simulink model "HVDCMTGW"  (R2025b)
settings: Solver=VariableStepAuto  StartTime=0.0  StopTime=Tsim  FixedStep=5e-5  RelTol=1e-3
PreLoadFcn:
  | SimulationTime = 3.5;
  | HVDCParameters;
  | Tsim = 3.5;
undefined symbols (not defined in the file): base, Base, Connection1, Connection2, Connection3, DiscIntNeverNeededParam, ee_sli_rtmsupport, frt, gcbh, grid, HVDC, lvrt, onshoreGfm, pll, pmsm, PVController, time, Ts, windController, windTransformer, windTurbine
libraries: fl_lib x51, ee_lib x46, nesl_utility x41, simulink x18, eeGeneralControl x12, eeTransforms x6
(part 4 of 4)

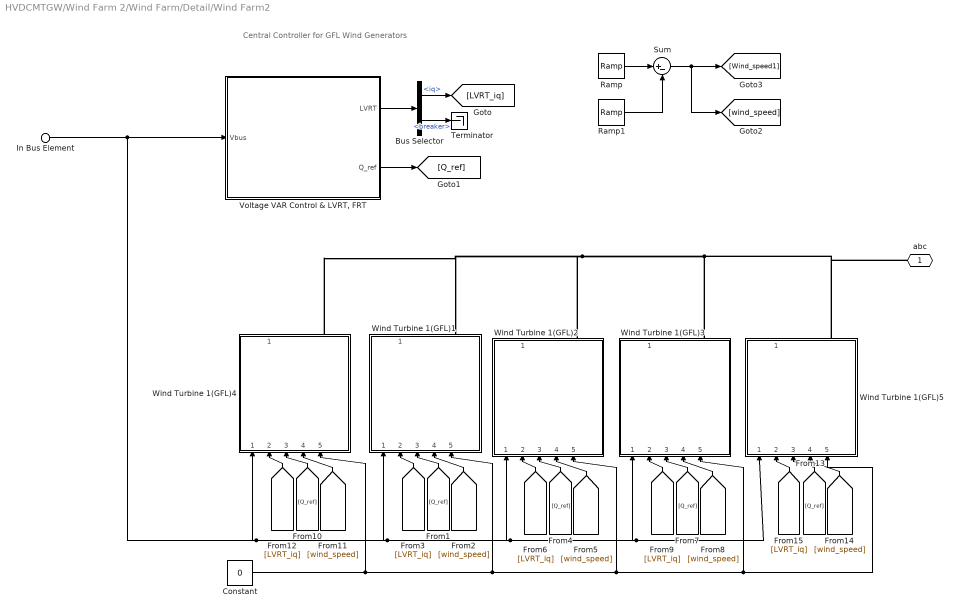
== system HVDCMTGW/Wind Farm 2/Wind Farm/Detail/Wind Farm2 ==
  note: Central Controller for GFL Wind Generators
  In Bus Element : Inport  PortName=Vbus
  Bus Selector : BusSelector  OutputSignals=iq,breaker
  Constant : Constant  Value=0
  Ramp : simulink/Sources/Ramp  slope=-3  start=time.renewablevariation  InitialOutput=11
  Ramp1 : simulink/Sources/Ramp  slope=-3  start=time.renewablevariation+0.2  InitialOutput=0
  Sum : Sum  Inputs=|+-
  Terminator : Terminator
  "Voltage VAR Control & LVRT, FRT" : Subsystem
      mask Display: image('$imagefile'); % Use "Edit Image" on toolstrip to change.
  Wind Turbine 1(GFL){1..5} (5 alike) : Subsystem  ReferencedSubsystem=WindGFLMpp  p=pmsm.p  psim=pmsm.psim  Rs=pmsm.rs  Ld=pmsm.ld  Lq=pmsm.lq  Kdip_sm=pmsm.ld*pmsm.alpha  Kdii_sm=pmsm.rs*pmsm.alpha  Kqip_sm=pmsm.lq*pmsm.alpha  Kqii_sm=pmsm.rs*pmsm.alpha  airDensity=windTurbine.airDensity  turbineRadius=windTurbine.turbineRadius  pitch=windTurbine.pitch  TSR=windTurbine.TSR  cp=windTurbine.cp  wt=0.01  rt=0.01  Inertia=windTurbine.inertia  Kp_dc=windController.kpv  Ki_dc=windController.kiv  Kdpi_g=windController.kpic  Kdii_g=windController.kiic  Kqpi_g=windController.kpic  Kqii_g=windController.kiic  blk=Enabled  slop=2  tst=0
  abc : PMIOPort  Side=Right
  wires:
  Bus Selector/2 -> Terminator/1  "<breaker>"
  "Voltage VAR Control & LVRT, FRT"/1(LVRT) -> Bus Selector/1
  Ramp1/1 -> Sum/2
  Ramp/1 -> Sum/1
  [LVRT_iq] -> Wind Turbine 1(GFL)1/2
  [wind_speed] -> Wind Turbine 1(GFL)1/4
  [Q_ref] -> Wind Turbine 1(GFL)1/3
  Sum/1 -> [Wind_speed1], [wind_speed]
  Bus Selector/1 -> [LVRT_iq]  "<iq>"
  "Voltage VAR Control & LVRT, FRT"/2(Q_ref) -> [Q_ref]
  [LVRT_iq] -> Wind Turbine 1(GFL)2/2
  [Q_ref] -> Wind Turbine 1(GFL)2/3
  [wind_speed] -> Wind Turbine 1(GFL)2/4
  [Q_ref] -> Wind Turbine 1(GFL)3/3
  [wind_speed] -> Wind Turbine 1(GFL)3/4
  [LVRT_iq] -> Wind Turbine 1(GFL)3/2
  In Bus Element/1 -> Wind Turbine 1(GFL)5/1, Wind Turbine 1(GFL)3/1, Wind Turbine 1(GFL)2/1, Wind Turbine 1(GFL)1/1, Wind Turbine 1(GFL)4/1, "Voltage VAR Control & LVRT, FRT"/1(Vbus)
  [LVRT_iq] -> Wind Turbine 1(GFL)4/2
  [Q_ref] -> Wind Turbine 1(GFL)4/3
  [wind_speed] -> Wind Turbine 1(GFL)4/4
  [LVRT_iq] -> Wind Turbine 1(GFL)5/2
  [Q_ref] -> Wind Turbine 1(GFL)5/3
  [wind_speed] -> Wind Turbine 1(GFL)5/4
  Constant/1 -> Wind Turbine 1(GFL)5/5, Wind Turbine 1(GFL)3/5, Wind Turbine 1(GFL)2/5, Wind Turbine 1(GFL)1/5, Wind Turbine 1(GFL)4/5
  connections:
  Wind Turbine 1(GFL)3/RConn1 -- abc/RConn1 -- Wind Turbine 1(GFL)5/RConn1 -- Wind Turbine 1(GFL)2/RConn1 -- Wind Turbine 1(GFL)4/RConn1 -- Wind Turbine 1(GFL)1/RConn1

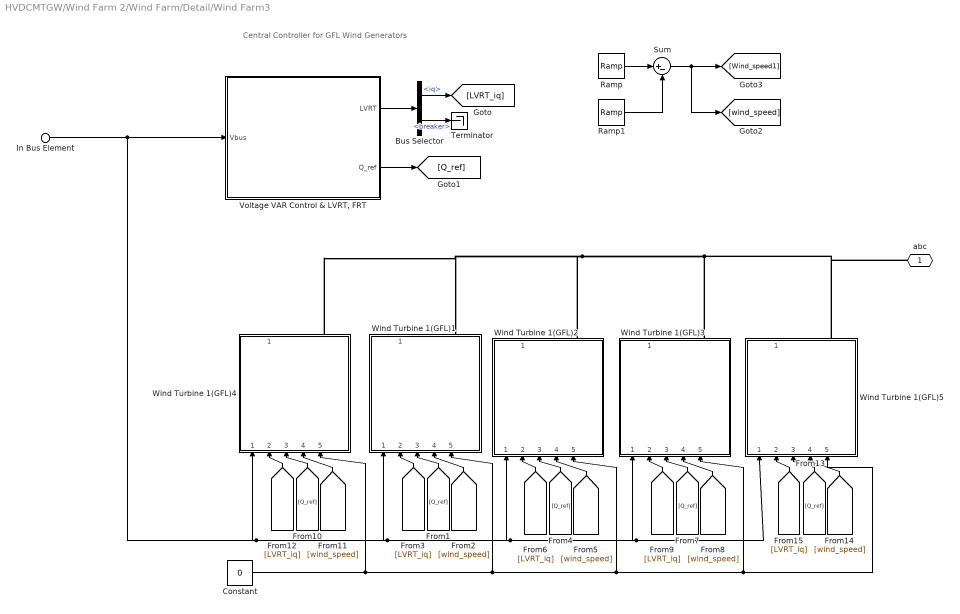
== system HVDCMTGW/Wind Farm 2/Wind Farm/Detail/Wind Farm3 ==
  note: Central Controller for GFL Wind Generators
  In Bus Element : Inport  PortName=Vbus
  Bus Selector : BusSelector  OutputSignals=iq,breaker
  Constant : Constant  Value=0
  Ramp : simulink/Sources/Ramp  slope=-3  start=time.renewablevariation  InitialOutput=11
  Ramp1 : simulink/Sources/Ramp  slope=-3  start=time.renewablevariation+0.2  InitialOutput=0
  Sum : Sum  Inputs=|+-
  Terminator : Terminator
  "Voltage VAR Control & LVRT, FRT" : Subsystem
      mask Display: image('$imagefile'); % Use "Edit Image" on toolstrip to change.
  Wind Turbine 1(GFL){1..5} (5 alike) : Subsystem  ReferencedSubsystem=WindGFLMpp  p=pmsm.p  psim=pmsm.psim  Rs=pmsm.rs  Ld=pmsm.ld  Lq=pmsm.lq  Kdip_sm=pmsm.ld*pmsm.alpha  Kdii_sm=pmsm.rs*pmsm.alpha  Kqip_sm=pmsm.lq*pmsm.alpha  Kqii_sm=pmsm.rs*pmsm.alpha  airDensity=windTurbine.airDensity  turbineRadius=windTurbine.turbineRadius  pitch=windTurbine.pitch  TSR=windTurbine.TSR  cp=windTurbine.cp  wt=0.01  rt=0.01  Inertia=windTurbine.inertia  Kp_dc=windController.kpv  Ki_dc=windController.kiv  Kdpi_g=windController.kpic  Kdii_g=windController.kiic  Kqpi_g=windController.kpic  Kqii_g=windController.kiic  blk=Enabled  slop=2  tst=0
  abc : PMIOPort  Side=Right
  wires:
  Bus Selector/2 -> Terminator/1  "<breaker>"
  "Voltage VAR Control & LVRT, FRT"/1(LVRT) -> Bus Selector/1
  Ramp1/1 -> Sum/2
  Ramp/1 -> Sum/1
  [LVRT_iq] -> Wind Turbine 1(GFL)1/2
  [wind_speed] -> Wind Turbine 1(GFL)1/4
  [Q_ref] -> Wind Turbine 1(GFL)1/3
  Sum/1 -> [Wind_speed1], [wind_speed]
  Bus Selector/1 -> [LVRT_iq]  "<iq>"
  "Voltage VAR Control & LVRT, FRT"/2(Q_ref) -> [Q_ref]
  [LVRT_iq] -> Wind Turbine 1(GFL)2/2
  [Q_ref] -> Wind Turbine 1(GFL)2/3
  [wind_speed] -> Wind Turbine 1(GFL)2/4
  [Q_ref] -> Wind Turbine 1(GFL)3/3
  [wind_speed] -> Wind Turbine 1(GFL)3/4
  [LVRT_iq] -> Wind Turbine 1(GFL)3/2
  In Bus Element/1 -> Wind Turbine 1(GFL)5/1, Wind Turbine 1(GFL)3/1, Wind Turbine 1(GFL)2/1, Wind Turbine 1(GFL)1/1, Wind Turbine 1(GFL)4/1, "Voltage VAR Control & LVRT, FRT"/1(Vbus)
  [LVRT_iq] -> Wind Turbine 1(GFL)4/2
  [Q_ref] -> Wind Turbine 1(GFL)4/3
  [wind_speed] -> Wind Turbine 1(GFL)4/4
  [LVRT_iq] -> Wind Turbine 1(GFL)5/2
  [Q_ref] -> Wind Turbine 1(GFL)5/3
  [wind_speed] -> Wind Turbine 1(GFL)5/4
  Constant/1 -> Wind Turbine 1(GFL)5/5, Wind Turbine 1(GFL)3/5, Wind Turbine 1(GFL)2/5, Wind Turbine 1(GFL)1/5, Wind Turbine 1(GFL)4/5
  connections:
  Wind Turbine 1(GFL)3/RConn1 -- abc/RConn1 -- Wind Turbine 1(GFL)5/RConn1 -- Wind Turbine 1(GFL)2/RConn1 -- Wind Turbine 1(GFL)4/RConn1 -- Wind Turbine 1(GFL)1/RConn1

== system HVDCMTGW/Wind Farm 1/PLL & Measurements/PLL/Sinusoidal Measurement (PLL, Three-Phase)1/Angle ==
  omega : Inport
  Integrator with Wrapped State (Discrete or Continuous) : eeGeneralControl/Integrator with Wrapped State (Discrete or Continuous)  LabelModeActiveChoice=Discrete  WrappedStateUpperValue=2*pi  WrappedStateLowerValue=0  x0=Theta0  Ts=Ts
      settings: LibrarySourceBlock=|
      | eeSinusoidalMeasurementV2/Sinusoidal Measurement
      | (PLL, Three-Phase)/Angle/Integrator with
      | Wrapped State
      | (Discrete or Continuous)
  theta : Outport  VectorParamsAs1DForOutWhenUnconnected=off
  wires:
  Integrator with Wrapped State (Discrete or Continuous)/1 -> theta/1
  omega/1 -> Integrator with Wrapped State (Discrete or Continuous)/1

== system HVDCMTGW/Wind Farm 1/PLL & Measurements/PLL/Sinusoidal Measurement (PLL, Three-Phase)1/PI ==
  u : Inport
  Constant : Constant  Value=2*pi*F0  SampleTime=Ts
  Constant1 : Constant  Value=0  SampleTime=Ts
  Data Type Conversion Inherited : simulink/Signal Attributes/Data Type Conversion Inherited  ConvertRealWorld=Real World Value  DoSatur=off
  Gain : Gain  Gain=Kp_LF
  Gain1 : Gain  Gain=Ki_LF
  Integrator (Discrete or Continuous) : eeGeneralControl/Integrator (Discrete or Continuous)  LabelModeActiveChoice=Discrete  IntegratorMethod=Integration: Forward Euler  ExternalReset=level  LimitType=Anti-windup  B=inf  A=-inf  Ts=Ts
      settings: LibrarySourceBlock=|
      | eeSinusoidalMeasurementV2/Sinusoidal Measurement
      | (PLL, Three-Phase)/PI/Integrator
      | (Discrete or Continuous)
  Sum : Sum  Inputs=|++
  y : Outport  VectorParamsAs1DForOutWhenUnconnected=off
  wires:
  Constant/1 -> Data Type Conversion Inherited/2
  Data Type Conversion Inherited/1 -> Integrator (Discrete or Continuous)/3
  Gain1/1 -> Integrator (Discrete or Continuous)/1
  u/1 -> Gain1/1, Data Type Conversion Inherited/1, Gain/1
  Gain/1 -> Sum/1
  Integrator (Discrete or Continuous)/1 -> Sum/2
  Sum/1 -> y/1
  Constant1/1 -> Integrator (Discrete or Continuous)/2

== system HVDCMTGW/Wind Farm 1/Wind Farm/Abstract/Wind Farm2/Voltage VAR Control & LVRT, FRT ==
  In Bus Element : Inport  PortName=Vbus  Element=Vmag
  In Bus Element1 : Inport  PortName=Vbus  Element=w
  Data Type Conversion : DataTypeConversion  RndMeth=Nearest  SaturateOnIntegerOverflow=off
  Delay : Delay  DelayLength=100
  Frequency RideThrough : Subsystem
  LVRT Characterstics : Subsystem
  OR : Logic  Operator=OR  IconShape=distinctive  AllPortsSameDT=off  OutDataTypeStr=boolean
  Unit Delay : UnitDelay  SampleTime=-1  HasFrameUpgradeWarning=on
  V_ref : Constant  Value=windController.vRef  SampleTime=Ts
  Voltage Control : Subsystem
  Out Bus Element : Outport  PortName=LVRT  Element=breaker
  Out Bus Element1 : Outport  PortName=LVRT  Element=iq
  Q_ref : Outport  Port=2
  wires:
  In Bus Element/1 -> LVRT Characterstics/1(Vmag), Voltage Control/1(In1)
  LVRT Characterstics/2(iq) -> Out Bus Element1/1
  V_ref/1 -> Voltage Control/2(In2)
  Voltage Control/1(Out1) -> Delay/1
  OR/1 -> Data Type Conversion/1
  LVRT Characterstics/1(Trip Signal) -> OR/1
  In Bus Element1/1 -> Frequency RideThrough/1(f)
  Data Type Conversion/1 -> Unit Delay/1
  Frequency RideThrough/1(Trip  Signal) -> OR/2
  Unit Delay/1 -> Out Bus Element/1
  Delay/1 -> Q_ref/1

== system HVDCMTGW/Wind Farm 1/Wind Farm/Detail/Wind Farm1/Voltage VAR Control & LVRT, FRT ==
  In Bus Element : Inport  PortName=Vbus  Element=Vmag
  In Bus Element1 : Inport  PortName=Vbus  Element=w
  Data Type Conversion : DataTypeConversion  RndMeth=Nearest  SaturateOnIntegerOverflow=off
  Delay : Delay  DelayLength=100
  Frequency RideThrough : Subsystem
  LVRT Characterstics : Subsystem
  OR : Logic  Operator=OR  IconShape=distinctive  AllPortsSameDT=off  OutDataTypeStr=boolean
  Unit Delay : UnitDelay  SampleTime=-1  HasFrameUpgradeWarning=on
  V_ref : Constant  Value=windController.vRef  SampleTime=Ts
  Voltage Control : Subsystem
  Out Bus Element : Outport  PortName=LVRT  Element=breaker
  Out Bus Element1 : Outport  PortName=LVRT  Element=iq
  Q_ref : Outport  Port=2
  wires:
  In Bus Element/1 -> LVRT Characterstics/1(Vmag), Voltage Control/1(In1)
  LVRT Characterstics/2(iq) -> Out Bus Element1/1
  V_ref/1 -> Voltage Control/2(In2)
  Voltage Control/1(Out1) -> Delay/1
  OR/1 -> Data Type Conversion/1
  LVRT Characterstics/1(Trip Signal) -> OR/1
  In Bus Element1/1 -> Frequency RideThrough/1(f)
  Data Type Conversion/1 -> Unit Delay/1
  Frequency RideThrough/1(Trip  Signal) -> OR/2
  Unit Delay/1 -> Out Bus Element/1
  Delay/1 -> Q_ref/1

== system HVDCMTGW/Wind Farm 1/Wind Farm/Detail/Wind Farm2/Voltage VAR Control & LVRT, FRT ==
  In Bus Element : Inport  PortName=Vbus  Element=Vmag
  In Bus Element1 : Inport  PortName=Vbus  Element=w
  Data Type Conversion : DataTypeConversion  RndMeth=Nearest  SaturateOnIntegerOverflow=off
  Delay : Delay  DelayLength=100
  Frequency RideThrough : Subsystem
  LVRT Characterstics : Subsystem
  OR : Logic  Operator=OR  IconShape=distinctive  AllPortsSameDT=off  OutDataTypeStr=boolean
  Unit Delay : UnitDelay  SampleTime=-1  HasFrameUpgradeWarning=on
  V_ref : Constant  Value=windController.vRef  SampleTime=Ts
  Voltage Control : Subsystem
  Out Bus Element : Outport  PortName=LVRT  Element=breaker
  Out Bus Element1 : Outport  PortName=LVRT  Element=iq
  Q_ref : Outport  Port=2
  wires:
  In Bus Element/1 -> LVRT Characterstics/1(Vmag), Voltage Control/1(In1)
  LVRT Characterstics/2(iq) -> Out Bus Element1/1
  V_ref/1 -> Voltage Control/2(In2)
  Voltage Control/1(Out1) -> Delay/1
  OR/1 -> Data Type Conversion/1
  LVRT Characterstics/1(Trip Signal) -> OR/1
  In Bus Element1/1 -> Frequency RideThrough/1(f)
  Data Type Conversion/1 -> Unit Delay/1
  Frequency RideThrough/1(Trip  Signal) -> OR/2
  Unit Delay/1 -> Out Bus Element/1
  Delay/1 -> Q_ref/1

== system HVDCMTGW/Wind Farm 1/Wind Farm/Detail/Wind Farm3/Voltage VAR Control & LVRT, FRT ==
  In Bus Element : Inport  PortName=Vbus  Element=Vmag
  In Bus Element1 : Inport  PortName=Vbus  Element=w
  Data Type Conversion : DataTypeConversion  RndMeth=Nearest  SaturateOnIntegerOverflow=off
  Delay : Delay  DelayLength=100
  Frequency RideThrough : Subsystem
  LVRT Characterstics : Subsystem
  OR : Logic  Operator=OR  IconShape=distinctive  AllPortsSameDT=off  OutDataTypeStr=boolean
  Unit Delay : UnitDelay  SampleTime=-1  HasFrameUpgradeWarning=on
  V_ref : Constant  Value=windController.vRef  SampleTime=Ts
  Voltage Control : Subsystem
  Out Bus Element : Outport  PortName=LVRT  Element=breaker
  Out Bus Element1 : Outport  PortName=LVRT  Element=iq
  Q_ref : Outport  Port=2
  wires:
  In Bus Element/1 -> LVRT Characterstics/1(Vmag), Voltage Control/1(In1)
  LVRT Characterstics/2(iq) -> Out Bus Element1/1
  V_ref/1 -> Voltage Control/2(In2)
  Voltage Control/1(Out1) -> Delay/1
  OR/1 -> Data Type Conversion/1
  LVRT Characterstics/1(Trip Signal) -> OR/1
  In Bus Element1/1 -> Frequency RideThrough/1(f)
  Data Type Conversion/1 -> Unit Delay/1
  Frequency RideThrough/1(Trip  Signal) -> OR/2
  Unit Delay/1 -> Out Bus Element/1
  Delay/1 -> Q_ref/1

== system HVDCMTGW/Wind Farm 2/PLL & Measurements/PLL/Sinusoidal Measurement (PLL, Three-Phase)1/Angle ==
  omega : Inport
  Integrator with Wrapped State (Discrete or Continuous) : eeGeneralControl/Integrator with Wrapped State (Discrete or Continuous)  LabelModeActiveChoice=Discrete  WrappedStateUpperValue=2*pi  WrappedStateLowerValue=0  x0=Theta0  Ts=Ts
      settings: LibrarySourceBlock=|
      | eeSinusoidalMeasurementV2/Sinusoidal Measurement
      | (PLL, Three-Phase)/Angle/Integrator with
      | Wrapped State
      | (Discrete or Continuous)
  theta : Outport  VectorParamsAs1DForOutWhenUnconnected=off
  wires:
  Integrator with Wrapped State (Discrete or Continuous)/1 -> theta/1
  omega/1 -> Integrator with Wrapped State (Discrete or Continuous)/1

== system HVDCMTGW/Wind Farm 2/PLL & Measurements/PLL/Sinusoidal Measurement (PLL, Three-Phase)1/PI ==
  u : Inport
  Constant : Constant  Value=2*pi*F0  SampleTime=Ts
  Constant1 : Constant  Value=0  SampleTime=Ts
  Data Type Conversion Inherited : simulink/Signal Attributes/Data Type Conversion Inherited  ConvertRealWorld=Real World Value  DoSatur=off
  Gain : Gain  Gain=Kp_LF
  Gain1 : Gain  Gain=Ki_LF
  Integrator (Discrete or Continuous) : eeGeneralControl/Integrator (Discrete or Continuous)  LabelModeActiveChoice=Discrete  IntegratorMethod=Integration: Forward Euler  ExternalReset=level  LimitType=Anti-windup  B=inf  A=-inf  Ts=Ts
      settings: LibrarySourceBlock=|
      | eeSinusoidalMeasurementV2/Sinusoidal Measurement
      | (PLL, Three-Phase)/PI/Integrator
      | (Discrete or Continuous)
  Sum : Sum  Inputs=|++
  y : Outport  VectorParamsAs1DForOutWhenUnconnected=off
  wires:
  Constant/1 -> Data Type Conversion Inherited/2
  Data Type Conversion Inherited/1 -> Integrator (Discrete or Continuous)/3
  Gain1/1 -> Integrator (Discrete or Continuous)/1
  u/1 -> Gain1/1, Data Type Conversion Inherited/1, Gain/1
  Gain/1 -> Sum/1
  Integrator (Discrete or Continuous)/1 -> Sum/2
  Sum/1 -> y/1
  Constant1/1 -> Integrator (Discrete or Continuous)/2

== system HVDCMTGW/Wind Farm 2/Wind Farm/Abstract/Wind Farm2/Voltage VAR Control & LVRT, FRT ==
  In Bus Element : Inport  PortName=Vbus  Element=Vmag
  In Bus Element1 : Inport  PortName=Vbus  Element=w
  Data Type Conversion : DataTypeConversion  RndMeth=Nearest  SaturateOnIntegerOverflow=off
  Delay : Delay  DelayLength=100
  Frequency RideThrough : Subsystem
  LVRT Characterstics : Subsystem
  OR : Logic  Operator=OR  IconShape=distinctive  AllPortsSameDT=off  OutDataTypeStr=boolean
  Unit Delay : UnitDelay  SampleTime=-1  HasFrameUpgradeWarning=on
  V_ref : Constant  Value=windController.vRef  SampleTime=Ts
  Voltage Control : Subsystem
  Out Bus Element : Outport  PortName=LVRT  Element=breaker
  Out Bus Element1 : Outport  PortName=LVRT  Element=iq
  Q_ref : Outport  Port=2
  wires:
  In Bus Element/1 -> LVRT Characterstics/1(Vmag), Voltage Control/1(In1)
  LVRT Characterstics/2(iq) -> Out Bus Element1/1
  V_ref/1 -> Voltage Control/2(In2)
  Voltage Control/1(Out1) -> Delay/1
  OR/1 -> Data Type Conversion/1
  LVRT Characterstics/1(Trip Signal) -> OR/1
  In Bus Element1/1 -> Frequency RideThrough/1(f)
  Data Type Conversion/1 -> Unit Delay/1
  Frequency RideThrough/1(Trip  Signal) -> OR/2
  Unit Delay/1 -> Out Bus Element/1
  Delay/1 -> Q_ref/1

== system HVDCMTGW/Wind Farm 2/Wind Farm/Detail/Wind Farm1/Voltage VAR Control & LVRT, FRT ==
  In Bus Element : Inport  PortName=Vbus  Element=Vmag
  In Bus Element1 : Inport  PortName=Vbus  Element=w
  Data Type Conversion : DataTypeConversion  RndMeth=Nearest  SaturateOnIntegerOverflow=off
  Delay : Delay  DelayLength=100
  Frequency RideThrough : Subsystem
  LVRT Characterstics : Subsystem
  OR : Logic  Operator=OR  IconShape=distinctive  AllPortsSameDT=off  OutDataTypeStr=boolean
  Unit Delay : UnitDelay  SampleTime=-1  HasFrameUpgradeWarning=on
  V_ref : Constant  Value=windController.vRef  SampleTime=Ts
  Voltage Control : Subsystem
  Out Bus Element : Outport  PortName=LVRT  Element=breaker
  Out Bus Element1 : Outport  PortName=LVRT  Element=iq
  Q_ref : Outport  Port=2
  wires:
  In Bus Element/1 -> LVRT Characterstics/1(Vmag), Voltage Control/1(In1)
  LVRT Characterstics/2(iq) -> Out Bus Element1/1
  V_ref/1 -> Voltage Control/2(In2)
  Voltage Control/1(Out1) -> Delay/1
  OR/1 -> Data Type Conversion/1
  LVRT Characterstics/1(Trip Signal) -> OR/1
  In Bus Element1/1 -> Frequency RideThrough/1(f)
  Data Type Conversion/1 -> Unit Delay/1
  Frequency RideThrough/1(Trip  Signal) -> OR/2
  Unit Delay/1 -> Out Bus Element/1
  Delay/1 -> Q_ref/1

== system HVDCMTGW/Wind Farm 2/Wind Farm/Detail/Wind Farm2/Voltage VAR Control & LVRT, FRT ==
  In Bus Element : Inport  PortName=Vbus  Element=Vmag
  In Bus Element1 : Inport  PortName=Vbus  Element=w
  Data Type Conversion : DataTypeConversion  RndMeth=Nearest  SaturateOnIntegerOverflow=off
  Delay : Delay  DelayLength=100
  Frequency RideThrough : Subsystem
  LVRT Characterstics : Subsystem
  OR : Logic  Operator=OR  IconShape=distinctive  AllPortsSameDT=off  OutDataTypeStr=boolean
  Unit Delay : UnitDelay  SampleTime=-1  HasFrameUpgradeWarning=on
  V_ref : Constant  Value=windController.vRef  SampleTime=Ts
  Voltage Control : Subsystem
  Out Bus Element : Outport  PortName=LVRT  Element=breaker
  Out Bus Element1 : Outport  PortName=LVRT  Element=iq
  Q_ref : Outport  Port=2
  wires:
  In Bus Element/1 -> LVRT Characterstics/1(Vmag), Voltage Control/1(In1)
  LVRT Characterstics/2(iq) -> Out Bus Element1/1
  V_ref/1 -> Voltage Control/2(In2)
  Voltage Control/1(Out1) -> Delay/1
  OR/1 -> Data Type Conversion/1
  LVRT Characterstics/1(Trip Signal) -> OR/1
  In Bus Element1/1 -> Frequency RideThrough/1(f)
  Data Type Conversion/1 -> Unit Delay/1
  Frequency RideThrough/1(Trip  Signal) -> OR/2
  Unit Delay/1 -> Out Bus Element/1
  Delay/1 -> Q_ref/1

== system HVDCMTGW/Wind Farm 2/Wind Farm/Detail/Wind Farm3/Voltage VAR Control & LVRT, FRT ==
  In Bus Element : Inport  PortName=Vbus  Element=Vmag
  In Bus Element1 : Inport  PortName=Vbus  Element=w
  Data Type Conversion : DataTypeConversion  RndMeth=Nearest  SaturateOnIntegerOverflow=off
  Delay : Delay  DelayLength=100
  Frequency RideThrough : Subsystem
  LVRT Characterstics : Subsystem
  OR : Logic  Operator=OR  IconShape=distinctive  AllPortsSameDT=off  OutDataTypeStr=boolean
  Unit Delay : UnitDelay  SampleTime=-1  HasFrameUpgradeWarning=on
  V_ref : Constant  Value=windController.vRef  SampleTime=Ts
  Voltage Control : Subsystem
  Out Bus Element : Outport  PortName=LVRT  Element=breaker
  Out Bus Element1 : Outport  PortName=LVRT  Element=iq
  Q_ref : Outport  Port=2
  wires:
  In Bus Element/1 -> LVRT Characterstics/1(Vmag), Voltage Control/1(In1)
  LVRT Characterstics/2(iq) -> Out Bus Element1/1
  V_ref/1 -> Voltage Control/2(In2)
  Voltage Control/1(Out1) -> Delay/1
  OR/1 -> Data Type Conversion/1
  LVRT Characterstics/1(Trip Signal) -> OR/1
  In Bus Element1/1 -> Frequency RideThrough/1(f)
  Data Type Conversion/1 -> Unit Delay/1
  Frequency RideThrough/1(Trip  Signal) -> OR/2
  Unit Delay/1 -> Out Bus Element/1
  Delay/1 -> Q_ref/1

== system HVDCMTGW/Wind Farm 1/Wind Farm/Abstract/Wind Farm2/Voltage VAR Control & LVRT, FRT/Frequency RideThrough ==
  f : Inport
  Avoid Operation : Subsystem
  Discrete-Time Integrator1 : DiscreteIntegrator  ExternalReset=either  SampleTime=Ts  ICPrevOutput=DiscIntNeverNeededParam  ICPrevScaledInput=DiscIntNeverNeededParam
  Duration of f<fth : Lookup_n-D  NumberOfTableDimensions=1  BreakpointsForDimension1=(1+[-0.021,-0.02,0.02,0.021])*grid.frequency  Table=[1,0,0,1]  InterpMethod=Flat  InternalRulePriority=Speed  RndMeth=Simplest
  Frequency vs Trip time : Lookup_n-D  NumberOfTableDimensions=1  BreakpointsForDimension1=frt.frequency  Table=frt.time  InterpMethod=Flat  InternalRulePriority=Speed  RndMeth=Simplest
  GreaterThan : RelationalOperator  Operator=>  OutDataTypeStr=boolean  RndMeth=Simplest  InputSameDT=off
  Trip  Signal : Outport
  wires:
  Discrete-Time Integrator1/1 -> GreaterThan/1
  Frequency vs Trip time/1 -> GreaterThan/2
  GreaterThan/1 -> Trip  Signal/1
  Duration of f<fth/1 -> Discrete-Time Integrator1/2, Discrete-Time Integrator1/1
  Avoid Operation/1(f) -> Duration of f<fth/1, Frequency vs Trip time/1
  f/1 -> Avoid Operation/1(f_in)

== system HVDCMTGW/Wind Farm 1/Wind Farm/Abstract/Wind Farm2/Voltage VAR Control & LVRT, FRT/LVRT Characterstics ==
  Vmag : Inport
  Discrete-Time Integrator1 : DiscreteIntegrator  ExternalReset=either  SampleTime=Ts  ICPrevOutput=DiscIntNeverNeededParam  ICPrevScaledInput=DiscIntNeverNeededParam
  Duration of Vmag<Vth : Lookup_n-D  NumberOfTableDimensions=1  BreakpointsForDimension1=[0,.9,0.91,1.2]  Table=[1,1,0,0]  InterpMethod=Flat  InternalRulePriority=Speed  RndMeth=Simplest
  Gain1 : Gain  Gain=-1
  GreaterThan : RelationalOperator  Operator=>  OutDataTypeStr=boolean  RndMeth=Simplest  InputSameDT=off
  Saturation2 : Saturate  UpperLimit=1/8  LowerLimit=-1
  Vmag vs Trip time : Lookup_n-D  NumberOfTableDimensions=1  BreakpointsForDimension1=lvrt.voltage  Table=lvrt.time  InterpMethod=Flat  InternalRulePriority=Speed  RndMeth=Simplest
  Vmag vs iq : Lookup_n-D  NumberOfTableDimensions=1  BreakpointsForDimension1=lvrt.voltageiq  Table=lvrt.iq  InternalRulePriority=Speed  RndMeth=Simplest
  Trip Signal : Outport
  iq : Outport  Port=2
  wires:
  Duration of Vmag<Vth/1 -> Discrete-Time Integrator1/2, Discrete-Time Integrator1/1
  GreaterThan/1 -> Trip Signal/1
  Discrete-Time Integrator1/1 -> GreaterThan/1
  Vmag vs Trip time/1 -> GreaterThan/2
  Vmag vs iq/1 -> Saturation2/1
  Gain1/1 -> iq/1
  Saturation2/1 -> Gain1/1
  Vmag/1 -> Vmag vs iq/1, Vmag vs Trip time/1, Duration of Vmag<Vth/1

== system HVDCMTGW/Wind Farm 1/Wind Farm/Abstract/Wind Farm2/Voltage VAR Control & LVRT, FRT/Voltage Control ==
  In1 : Inport
  In2 : Inport  Port=2
  Constant2 : Constant  Value=0
  Gain : Gain  Gain=windController.mv
  Sum2 : Sum  Inputs=|+-
  Switch1 : Switch  Threshold=.9  SaturateOnIntegerOverflow=off  InputSameDT=off
  Out1 : Outport
  wires:
  Gain/1 -> Out1/1
  Sum2/1 -> Switch1/1
  Switch1/1 -> Gain/1
  In1/1 -> Sum2/2, Switch1/2
  Constant2/1 -> Switch1/3
  In2/1 -> Sum2/1

== system HVDCMTGW/Wind Farm 1/Wind Farm/Detail/Wind Farm1/Voltage VAR Control & LVRT, FRT/Frequency RideThrough ==
  f : Inport
  Avoid Operation : Subsystem
  Discrete-Time Integrator1 : DiscreteIntegrator  ExternalReset=either  SampleTime=Ts  ICPrevOutput=DiscIntNeverNeededParam  ICPrevScaledInput=DiscIntNeverNeededParam
  Duration of f<fth : Lookup_n-D  NumberOfTableDimensions=1  BreakpointsForDimension1=(1+[-0.021,-0.02,0.02,0.021])*grid.frequency  Table=[1,0,0,1]  InterpMethod=Flat  InternalRulePriority=Speed  RndMeth=Simplest
  Frequency vs Trip time : Lookup_n-D  NumberOfTableDimensions=1  BreakpointsForDimension1=frt.frequency  Table=frt.time  InterpMethod=Flat  InternalRulePriority=Speed  RndMeth=Simplest
  GreaterThan : RelationalOperator  Operator=>  OutDataTypeStr=boolean  RndMeth=Simplest  InputSameDT=off
  Trip  Signal : Outport
  wires:
  Discrete-Time Integrator1/1 -> GreaterThan/1
  Frequency vs Trip time/1 -> GreaterThan/2
  GreaterThan/1 -> Trip  Signal/1
  Duration of f<fth/1 -> Discrete-Time Integrator1/2, Discrete-Time Integrator1/1
  Avoid Operation/1(f) -> Duration of f<fth/1, Frequency vs Trip time/1
  f/1 -> Avoid Operation/1(f_in)

== system HVDCMTGW/Wind Farm 1/Wind Farm/Detail/Wind Farm1/Voltage VAR Control & LVRT, FRT/LVRT Characterstics ==
  Vmag : Inport
  Discrete-Time Integrator1 : DiscreteIntegrator  ExternalReset=either  SampleTime=Ts  ICPrevOutput=DiscIntNeverNeededParam  ICPrevScaledInput=DiscIntNeverNeededParam
  Duration of Vmag<Vth : Lookup_n-D  NumberOfTableDimensions=1  BreakpointsForDimension1=[0,.9,0.91,1.2]  Table=[1,1,0,0]  InterpMethod=Flat  InternalRulePriority=Speed  RndMeth=Simplest
  Gain1 : Gain  Gain=-1
  GreaterThan : RelationalOperator  Operator=>  OutDataTypeStr=boolean  RndMeth=Simplest  InputSameDT=off
  Saturation2 : Saturate  UpperLimit=1/8  LowerLimit=-1
  Vmag vs Trip time : Lookup_n-D  NumberOfTableDimensions=1  BreakpointsForDimension1=lvrt.voltage  Table=lvrt.time  InterpMethod=Flat  InternalRulePriority=Speed  RndMeth=Simplest
  Vmag vs iq : Lookup_n-D  NumberOfTableDimensions=1  BreakpointsForDimension1=lvrt.voltageiq  Table=lvrt.iq  InternalRulePriority=Speed  RndMeth=Simplest
  Trip Signal : Outport
  iq : Outport  Port=2
  wires:
  Duration of Vmag<Vth/1 -> Discrete-Time Integrator1/2, Discrete-Time Integrator1/1
  GreaterThan/1 -> Trip Signal/1
  Discrete-Time Integrator1/1 -> GreaterThan/1
  Vmag vs Trip time/1 -> GreaterThan/2
  Vmag vs iq/1 -> Saturation2/1
  Gain1/1 -> iq/1
  Saturation2/1 -> Gain1/1
  Vmag/1 -> Vmag vs iq/1, Vmag vs Trip time/1, Duration of Vmag<Vth/1

== system HVDCMTGW/Wind Farm 1/Wind Farm/Detail/Wind Farm1/Voltage VAR Control & LVRT, FRT/Voltage Control ==
  In1 : Inport
  In2 : Inport  Port=2
  Constant2 : Constant  Value=0
  Gain : Gain  Gain=windController.mv
  Sum2 : Sum  Inputs=|+-
  Switch1 : Switch  Threshold=.9  SaturateOnIntegerOverflow=off  InputSameDT=off
  Out1 : Outport
  wires:
  Gain/1 -> Out1/1
  Sum2/1 -> Switch1/1
  Switch1/1 -> Gain/1
  In1/1 -> Sum2/2, Switch1/2
  Constant2/1 -> Switch1/3
  In2/1 -> Sum2/1

== system HVDCMTGW/Wind Farm 1/Wind Farm/Detail/Wind Farm2/Voltage VAR Control & LVRT, FRT/Frequency RideThrough ==
  f : Inport
  Avoid Operation : Subsystem
  Discrete-Time Integrator1 : DiscreteIntegrator  ExternalReset=either  SampleTime=Ts  ICPrevOutput=DiscIntNeverNeededParam  ICPrevScaledInput=DiscIntNeverNeededParam
  Duration of f<fth : Lookup_n-D  NumberOfTableDimensions=1  BreakpointsForDimension1=(1+[-0.021,-0.02,0.02,0.021])*grid.frequency  Table=[1,0,0,1]  InterpMethod=Flat  InternalRulePriority=Speed  RndMeth=Simplest
  Frequency vs Trip time : Lookup_n-D  NumberOfTableDimensions=1  BreakpointsForDimension1=frt.frequency  Table=frt.time  InterpMethod=Flat  InternalRulePriority=Speed  RndMeth=Simplest
  GreaterThan : RelationalOperator  Operator=>  OutDataTypeStr=boolean  RndMeth=Simplest  InputSameDT=off
  Trip  Signal : Outport
  wires:
  Discrete-Time Integrator1/1 -> GreaterThan/1
  Frequency vs Trip time/1 -> GreaterThan/2
  GreaterThan/1 -> Trip  Signal/1
  Duration of f<fth/1 -> Discrete-Time Integrator1/2, Discrete-Time Integrator1/1
  Avoid Operation/1(f) -> Duration of f<fth/1, Frequency vs Trip time/1
  f/1 -> Avoid Operation/1(f_in)

== system HVDCMTGW/Wind Farm 1/Wind Farm/Detail/Wind Farm2/Voltage VAR Control & LVRT, FRT/LVRT Characterstics ==
  Vmag : Inport
  Discrete-Time Integrator1 : DiscreteIntegrator  ExternalReset=either  SampleTime=Ts  ICPrevOutput=DiscIntNeverNeededParam  ICPrevScaledInput=DiscIntNeverNeededParam
  Duration of Vmag<Vth : Lookup_n-D  NumberOfTableDimensions=1  BreakpointsForDimension1=[0,.9,0.91,1.2]  Table=[1,1,0,0]  InterpMethod=Flat  InternalRulePriority=Speed  RndMeth=Simplest
  Gain1 : Gain  Gain=-1
  GreaterThan : RelationalOperator  Operator=>  OutDataTypeStr=boolean  RndMeth=Simplest  InputSameDT=off
  Saturation2 : Saturate  UpperLimit=1/8  LowerLimit=-1
  Vmag vs Trip time : Lookup_n-D  NumberOfTableDimensions=1  BreakpointsForDimension1=lvrt.voltage  Table=lvrt.time  InterpMethod=Flat  InternalRulePriority=Speed  RndMeth=Simplest
  Vmag vs iq : Lookup_n-D  NumberOfTableDimensions=1  BreakpointsForDimension1=lvrt.voltageiq  Table=lvrt.iq  InternalRulePriority=Speed  RndMeth=Simplest
  Trip Signal : Outport
  iq : Outport  Port=2
  wires:
  Duration of Vmag<Vth/1 -> Discrete-Time Integrator1/2, Discrete-Time Integrator1/1
  GreaterThan/1 -> Trip Signal/1
  Discrete-Time Integrator1/1 -> GreaterThan/1
  Vmag vs Trip time/1 -> GreaterThan/2
  Vmag vs iq/1 -> Saturation2/1
  Gain1/1 -> iq/1
  Saturation2/1 -> Gain1/1
  Vmag/1 -> Vmag vs iq/1, Vmag vs Trip time/1, Duration of Vmag<Vth/1

== system HVDCMTGW/Wind Farm 1/Wind Farm/Detail/Wind Farm2/Voltage VAR Control & LVRT, FRT/Voltage Control ==
  In1 : Inport
  In2 : Inport  Port=2
  Constant2 : Constant  Value=0
  Gain : Gain  Gain=windController.mv
  Sum2 : Sum  Inputs=|+-
  Switch1 : Switch  Threshold=.9  SaturateOnIntegerOverflow=off  InputSameDT=off
  Out1 : Outport
  wires:
  Gain/1 -> Out1/1
  Sum2/1 -> Switch1/1
  Switch1/1 -> Gain/1
  In1/1 -> Sum2/2, Switch1/2
  Constant2/1 -> Switch1/3
  In2/1 -> Sum2/1

== system HVDCMTGW/Wind Farm 1/Wind Farm/Detail/Wind Farm3/Voltage VAR Control & LVRT, FRT/Frequency RideThrough ==
  f : Inport
  Avoid Operation : Subsystem
  Discrete-Time Integrator1 : DiscreteIntegrator  ExternalReset=either  SampleTime=Ts  ICPrevOutput=DiscIntNeverNeededParam  ICPrevScaledInput=DiscIntNeverNeededParam
  Duration of f<fth : Lookup_n-D  NumberOfTableDimensions=1  BreakpointsForDimension1=(1+[-0.021,-0.02,0.02,0.021])*grid.frequency  Table=[1,0,0,1]  InterpMethod=Flat  InternalRulePriority=Speed  RndMeth=Simplest
  Frequency vs Trip time : Lookup_n-D  NumberOfTableDimensions=1  BreakpointsForDimension1=frt.frequency  Table=frt.time  InterpMethod=Flat  InternalRulePriority=Speed  RndMeth=Simplest
  GreaterThan : RelationalOperator  Operator=>  OutDataTypeStr=boolean  RndMeth=Simplest  InputSameDT=off
  Trip  Signal : Outport
  wires:
  Discrete-Time Integrator1/1 -> GreaterThan/1
  Frequency vs Trip time/1 -> GreaterThan/2
  GreaterThan/1 -> Trip  Signal/1
  Duration of f<fth/1 -> Discrete-Time Integrator1/2, Discrete-Time Integrator1/1
  Avoid Operation/1(f) -> Duration of f<fth/1, Frequency vs Trip time/1
  f/1 -> Avoid Operation/1(f_in)

== system HVDCMTGW/Wind Farm 1/Wind Farm/Detail/Wind Farm3/Voltage VAR Control & LVRT, FRT/LVRT Characterstics ==
  Vmag : Inport
  Discrete-Time Integrator1 : DiscreteIntegrator  ExternalReset=either  SampleTime=Ts  ICPrevOutput=DiscIntNeverNeededParam  ICPrevScaledInput=DiscIntNeverNeededParam
  Duration of Vmag<Vth : Lookup_n-D  NumberOfTableDimensions=1  BreakpointsForDimension1=[0,.9,0.91,1.2]  Table=[1,1,0,0]  InterpMethod=Flat  InternalRulePriority=Speed  RndMeth=Simplest
  Gain1 : Gain  Gain=-1
  GreaterThan : RelationalOperator  Operator=>  OutDataTypeStr=boolean  RndMeth=Simplest  InputSameDT=off
  Saturation2 : Saturate  UpperLimit=1/8  LowerLimit=-1
  Vmag vs Trip time : Lookup_n-D  NumberOfTableDimensions=1  BreakpointsForDimension1=lvrt.voltage  Table=lvrt.time  InterpMethod=Flat  InternalRulePriority=Speed  RndMeth=Simplest
  Vmag vs iq : Lookup_n-D  NumberOfTableDimensions=1  BreakpointsForDimension1=lvrt.voltageiq  Table=lvrt.iq  InternalRulePriority=Speed  RndMeth=Simplest
  Trip Signal : Outport
  iq : Outport  Port=2
  wires:
  Duration of Vmag<Vth/1 -> Discrete-Time Integrator1/2, Discrete-Time Integrator1/1
  GreaterThan/1 -> Trip Signal/1
  Discrete-Time Integrator1/1 -> GreaterThan/1
  Vmag vs Trip time/1 -> GreaterThan/2
  Vmag vs iq/1 -> Saturation2/1
  Gain1/1 -> iq/1
  Saturation2/1 -> Gain1/1
  Vmag/1 -> Vmag vs iq/1, Vmag vs Trip time/1, Duration of Vmag<Vth/1

== system HVDCMTGW/Wind Farm 1/Wind Farm/Detail/Wind Farm3/Voltage VAR Control & LVRT, FRT/Voltage Control ==
  In1 : Inport
  In2 : Inport  Port=2
  Constant2 : Constant  Value=0
  Gain : Gain  Gain=windController.mv
  Sum2 : Sum  Inputs=|+-
  Switch1 : Switch  Threshold=.9  SaturateOnIntegerOverflow=off  InputSameDT=off
  Out1 : Outport
  wires:
  Gain/1 -> Out1/1
  Sum2/1 -> Switch1/1
  Switch1/1 -> Gain/1
  In1/1 -> Sum2/2, Switch1/2
  Constant2/1 -> Switch1/3
  In2/1 -> Sum2/1

== system HVDCMTGW/Wind Farm 2/Wind Farm/Abstract/Wind Farm2/Voltage VAR Control & LVRT, FRT/Frequency RideThrough ==
  f : Inport
  Avoid Operation : Subsystem
  Discrete-Time Integrator1 : DiscreteIntegrator  ExternalReset=either  SampleTime=Ts  ICPrevOutput=DiscIntNeverNeededParam  ICPrevScaledInput=DiscIntNeverNeededParam
  Duration of f<fth : Lookup_n-D  NumberOfTableDimensions=1  BreakpointsForDimension1=(1+[-0.021,-0.02,0.02,0.021])*grid.frequency  Table=[1,0,0,1]  InterpMethod=Flat  InternalRulePriority=Speed  RndMeth=Simplest
  Frequency vs Trip time : Lookup_n-D  NumberOfTableDimensions=1  BreakpointsForDimension1=frt.frequency  Table=frt.time  InterpMethod=Flat  InternalRulePriority=Speed  RndMeth=Simplest
  GreaterThan : RelationalOperator  Operator=>  OutDataTypeStr=boolean  RndMeth=Simplest  InputSameDT=off
  Trip  Signal : Outport
  wires:
  Discrete-Time Integrator1/1 -> GreaterThan/1
  Frequency vs Trip time/1 -> GreaterThan/2
  GreaterThan/1 -> Trip  Signal/1
  Duration of f<fth/1 -> Discrete-Time Integrator1/2, Discrete-Time Integrator1/1
  Avoid Operation/1(f) -> Duration of f<fth/1, Frequency vs Trip time/1
  f/1 -> Avoid Operation/1(f_in)

== system HVDCMTGW/Wind Farm 2/Wind Farm/Abstract/Wind Farm2/Voltage VAR Control & LVRT, FRT/LVRT Characterstics ==
  Vmag : Inport
  Discrete-Time Integrator1 : DiscreteIntegrator  ExternalReset=either  SampleTime=Ts  ICPrevOutput=DiscIntNeverNeededParam  ICPrevScaledInput=DiscIntNeverNeededParam
  Duration of Vmag<Vth : Lookup_n-D  NumberOfTableDimensions=1  BreakpointsForDimension1=[0,.9,0.91,1.2]  Table=[1,1,0,0]  InterpMethod=Flat  InternalRulePriority=Speed  RndMeth=Simplest
  Gain1 : Gain  Gain=-1
  GreaterThan : RelationalOperator  Operator=>  OutDataTypeStr=boolean  RndMeth=Simplest  InputSameDT=off
  Saturation2 : Saturate  UpperLimit=1/8  LowerLimit=-1
  Vmag vs Trip time : Lookup_n-D  NumberOfTableDimensions=1  BreakpointsForDimension1=lvrt.voltage  Table=lvrt.time  InterpMethod=Flat  InternalRulePriority=Speed  RndMeth=Simplest
  Vmag vs iq : Lookup_n-D  NumberOfTableDimensions=1  BreakpointsForDimension1=lvrt.voltageiq  Table=lvrt.iq  InternalRulePriority=Speed  RndMeth=Simplest
  Trip Signal : Outport
  iq : Outport  Port=2
  wires:
  Duration of Vmag<Vth/1 -> Discrete-Time Integrator1/2, Discrete-Time Integrator1/1
  GreaterThan/1 -> Trip Signal/1
  Discrete-Time Integrator1/1 -> GreaterThan/1
  Vmag vs Trip time/1 -> GreaterThan/2
  Vmag vs iq/1 -> Saturation2/1
  Gain1/1 -> iq/1
  Saturation2/1 -> Gain1/1
  Vmag/1 -> Vmag vs iq/1, Vmag vs Trip time/1, Duration of Vmag<Vth/1

== system HVDCMTGW/Wind Farm 2/Wind Farm/Abstract/Wind Farm2/Voltage VAR Control & LVRT, FRT/Voltage Control ==
  In1 : Inport
  In2 : Inport  Port=2
  Constant2 : Constant  Value=0
  Gain : Gain  Gain=windController.mv
  Sum2 : Sum  Inputs=|+-
  Switch1 : Switch  Threshold=.9  SaturateOnIntegerOverflow=off  InputSameDT=off
  Out1 : Outport
  wires:
  Gain/1 -> Out1/1
  Sum2/1 -> Switch1/1
  Switch1/1 -> Gain/1
  In1/1 -> Sum2/2, Switch1/2
  Constant2/1 -> Switch1/3
  In2/1 -> Sum2/1

== system HVDCMTGW/Wind Farm 2/Wind Farm/Detail/Wind Farm1/Voltage VAR Control & LVRT, FRT/Frequency RideThrough ==
  f : Inport
  Avoid Operation : Subsystem
  Discrete-Time Integrator1 : DiscreteIntegrator  ExternalReset=either  SampleTime=Ts  ICPrevOutput=DiscIntNeverNeededParam  ICPrevScaledInput=DiscIntNeverNeededParam
  Duration of f<fth : Lookup_n-D  NumberOfTableDimensions=1  BreakpointsForDimension1=(1+[-0.021,-0.02,0.02,0.021])*grid.frequency  Table=[1,0,0,1]  InterpMethod=Flat  InternalRulePriority=Speed  RndMeth=Simplest
  Frequency vs Trip time : Lookup_n-D  NumberOfTableDimensions=1  BreakpointsForDimension1=frt.frequency  Table=frt.time  InterpMethod=Flat  InternalRulePriority=Speed  RndMeth=Simplest
  GreaterThan : RelationalOperator  Operator=>  OutDataTypeStr=boolean  RndMeth=Simplest  InputSameDT=off
  Trip  Signal : Outport
  wires:
  Discrete-Time Integrator1/1 -> GreaterThan/1
  Frequency vs Trip time/1 -> GreaterThan/2
  GreaterThan/1 -> Trip  Signal/1
  Duration of f<fth/1 -> Discrete-Time Integrator1/2, Discrete-Time Integrator1/1
  Avoid Operation/1(f) -> Duration of f<fth/1, Frequency vs Trip time/1
  f/1 -> Avoid Operation/1(f_in)

== system HVDCMTGW/Wind Farm 2/Wind Farm/Detail/Wind Farm1/Voltage VAR Control & LVRT, FRT/LVRT Characterstics ==
  Vmag : Inport
  Discrete-Time Integrator1 : DiscreteIntegrator  ExternalReset=either  SampleTime=Ts  ICPrevOutput=DiscIntNeverNeededParam  ICPrevScaledInput=DiscIntNeverNeededParam
  Duration of Vmag<Vth : Lookup_n-D  NumberOfTableDimensions=1  BreakpointsForDimension1=[0,.9,0.91,1.2]  Table=[1,1,0,0]  InterpMethod=Flat  InternalRulePriority=Speed  RndMeth=Simplest
  Gain1 : Gain  Gain=-1
  GreaterThan : RelationalOperator  Operator=>  OutDataTypeStr=boolean  RndMeth=Simplest  InputSameDT=off
  Saturation2 : Saturate  UpperLimit=1/8  LowerLimit=-1
  Vmag vs Trip time : Lookup_n-D  NumberOfTableDimensions=1  BreakpointsForDimension1=lvrt.voltage  Table=lvrt.time  InterpMethod=Flat  InternalRulePriority=Speed  RndMeth=Simplest
  Vmag vs iq : Lookup_n-D  NumberOfTableDimensions=1  BreakpointsForDimension1=lvrt.voltageiq  Table=lvrt.iq  InternalRulePriority=Speed  RndMeth=Simplest
  Trip Signal : Outport
  iq : Outport  Port=2
  wires:
  Duration of Vmag<Vth/1 -> Discrete-Time Integrator1/2, Discrete-Time Integrator1/1
  GreaterThan/1 -> Trip Signal/1
  Discrete-Time Integrator1/1 -> GreaterThan/1
  Vmag vs Trip time/1 -> GreaterThan/2
  Vmag vs iq/1 -> Saturation2/1
  Gain1/1 -> iq/1
  Saturation2/1 -> Gain1/1
  Vmag/1 -> Vmag vs iq/1, Vmag vs Trip time/1, Duration of Vmag<Vth/1

== system HVDCMTGW/Wind Farm 2/Wind Farm/Detail/Wind Farm1/Voltage VAR Control & LVRT, FRT/Voltage Control ==
  In1 : Inport
  In2 : Inport  Port=2
  Constant2 : Constant  Value=0
  Gain : Gain  Gain=windController.mv
  Sum2 : Sum  Inputs=|+-
  Switch1 : Switch  Threshold=.9  SaturateOnIntegerOverflow=off  InputSameDT=off
  Out1 : Outport
  wires:
  Gain/1 -> Out1/1
  Sum2/1 -> Switch1/1
  Switch1/1 -> Gain/1
  In1/1 -> Sum2/2, Switch1/2
  Constant2/1 -> Switch1/3
  In2/1 -> Sum2/1

== system HVDCMTGW/Wind Farm 2/Wind Farm/Detail/Wind Farm2/Voltage VAR Control & LVRT, FRT/Frequency RideThrough ==
  f : Inport
  Avoid Operation : Subsystem
  Discrete-Time Integrator1 : DiscreteIntegrator  ExternalReset=either  SampleTime=Ts  ICPrevOutput=DiscIntNeverNeededParam  ICPrevScaledInput=DiscIntNeverNeededParam
  Duration of f<fth : Lookup_n-D  NumberOfTableDimensions=1  BreakpointsForDimension1=(1+[-0.021,-0.02,0.02,0.021])*grid.frequency  Table=[1,0,0,1]  InterpMethod=Flat  InternalRulePriority=Speed  RndMeth=Simplest
  Frequency vs Trip time : Lookup_n-D  NumberOfTableDimensions=1  BreakpointsForDimension1=frt.frequency  Table=frt.time  InterpMethod=Flat  InternalRulePriority=Speed  RndMeth=Simplest
  GreaterThan : RelationalOperator  Operator=>  OutDataTypeStr=boolean  RndMeth=Simplest  InputSameDT=off
  Trip  Signal : Outport
  wires:
  Discrete-Time Integrator1/1 -> GreaterThan/1
  Frequency vs Trip time/1 -> GreaterThan/2
  GreaterThan/1 -> Trip  Signal/1
  Duration of f<fth/1 -> Discrete-Time Integrator1/2, Discrete-Time Integrator1/1
  Avoid Operation/1(f) -> Duration of f<fth/1, Frequency vs Trip time/1
  f/1 -> Avoid Operation/1(f_in)

== system HVDCMTGW/Wind Farm 2/Wind Farm/Detail/Wind Farm2/Voltage VAR Control & LVRT, FRT/LVRT Characterstics ==
  Vmag : Inport
  Discrete-Time Integrator1 : DiscreteIntegrator  ExternalReset=either  SampleTime=Ts  ICPrevOutput=DiscIntNeverNeededParam  ICPrevScaledInput=DiscIntNeverNeededParam
  Duration of Vmag<Vth : Lookup_n-D  NumberOfTableDimensions=1  BreakpointsForDimension1=[0,.9,0.91,1.2]  Table=[1,1,0,0]  InterpMethod=Flat  InternalRulePriority=Speed  RndMeth=Simplest
  Gain1 : Gain  Gain=-1
  GreaterThan : RelationalOperator  Operator=>  OutDataTypeStr=boolean  RndMeth=Simplest  InputSameDT=off
  Saturation2 : Saturate  UpperLimit=1/8  LowerLimit=-1
  Vmag vs Trip time : Lookup_n-D  NumberOfTableDimensions=1  BreakpointsForDimension1=lvrt.voltage  Table=lvrt.time  InterpMethod=Flat  InternalRulePriority=Speed  RndMeth=Simplest
  Vmag vs iq : Lookup_n-D  NumberOfTableDimensions=1  BreakpointsForDimension1=lvrt.voltageiq  Table=lvrt.iq  InternalRulePriority=Speed  RndMeth=Simplest
  Trip Signal : Outport
  iq : Outport  Port=2
  wires:
  Duration of Vmag<Vth/1 -> Discrete-Time Integrator1/2, Discrete-Time Integrator1/1
  GreaterThan/1 -> Trip Signal/1
  Discrete-Time Integrator1/1 -> GreaterThan/1
  Vmag vs Trip time/1 -> GreaterThan/2
  Vmag vs iq/1 -> Saturation2/1
  Gain1/1 -> iq/1
  Saturation2/1 -> Gain1/1
  Vmag/1 -> Vmag vs iq/1, Vmag vs Trip time/1, Duration of Vmag<Vth/1

== system HVDCMTGW/Wind Farm 2/Wind Farm/Detail/Wind Farm2/Voltage VAR Control & LVRT, FRT/Voltage Control ==
  In1 : Inport
  In2 : Inport  Port=2
  Constant2 : Constant  Value=0
  Gain : Gain  Gain=windController.mv
  Sum2 : Sum  Inputs=|+-
  Switch1 : Switch  Threshold=.9  SaturateOnIntegerOverflow=off  InputSameDT=off
  Out1 : Outport
  wires:
  Gain/1 -> Out1/1
  Sum2/1 -> Switch1/1
  Switch1/1 -> Gain/1
  In1/1 -> Sum2/2, Switch1/2
  Constant2/1 -> Switch1/3
  In2/1 -> Sum2/1

== system HVDCMTGW/Wind Farm 2/Wind Farm/Detail/Wind Farm3/Voltage VAR Control & LVRT, FRT/Frequency RideThrough ==
  f : Inport
  Avoid Operation : Subsystem
  Discrete-Time Integrator1 : DiscreteIntegrator  ExternalReset=either  SampleTime=Ts  ICPrevOutput=DiscIntNeverNeededParam  ICPrevScaledInput=DiscIntNeverNeededParam
  Duration of f<fth : Lookup_n-D  NumberOfTableDimensions=1  BreakpointsForDimension1=(1+[-0.021,-0.02,0.02,0.021])*grid.frequency  Table=[1,0,0,1]  InterpMethod=Flat  InternalRulePriority=Speed  RndMeth=Simplest
  Frequency vs Trip time : Lookup_n-D  NumberOfTableDimensions=1  BreakpointsForDimension1=frt.frequency  Table=frt.time  InterpMethod=Flat  InternalRulePriority=Speed  RndMeth=Simplest
  GreaterThan : RelationalOperator  Operator=>  OutDataTypeStr=boolean  RndMeth=Simplest  InputSameDT=off
  Trip  Signal : Outport
  wires:
  Discrete-Time Integrator1/1 -> GreaterThan/1
  Frequency vs Trip time/1 -> GreaterThan/2
  GreaterThan/1 -> Trip  Signal/1
  Duration of f<fth/1 -> Discrete-Time Integrator1/2, Discrete-Time Integrator1/1
  Avoid Operation/1(f) -> Duration of f<fth/1, Frequency vs Trip time/1
  f/1 -> Avoid Operation/1(f_in)

== system HVDCMTGW/Wind Farm 2/Wind Farm/Detail/Wind Farm3/Voltage VAR Control & LVRT, FRT/LVRT Characterstics ==
  Vmag : Inport
  Discrete-Time Integrator1 : DiscreteIntegrator  ExternalReset=either  SampleTime=Ts  ICPrevOutput=DiscIntNeverNeededParam  ICPrevScaledInput=DiscIntNeverNeededParam
  Duration of Vmag<Vth : Lookup_n-D  NumberOfTableDimensions=1  BreakpointsForDimension1=[0,.9,0.91,1.2]  Table=[1,1,0,0]  InterpMethod=Flat  InternalRulePriority=Speed  RndMeth=Simplest
  Gain1 : Gain  Gain=-1
  GreaterThan : RelationalOperator  Operator=>  OutDataTypeStr=boolean  RndMeth=Simplest  InputSameDT=off
  Saturation2 : Saturate  UpperLimit=1/8  LowerLimit=-1
  Vmag vs Trip time : Lookup_n-D  NumberOfTableDimensions=1  BreakpointsForDimension1=lvrt.voltage  Table=lvrt.time  InterpMethod=Flat  InternalRulePriority=Speed  RndMeth=Simplest
  Vmag vs iq : Lookup_n-D  NumberOfTableDimensions=1  BreakpointsForDimension1=lvrt.voltageiq  Table=lvrt.iq  InternalRulePriority=Speed  RndMeth=Simplest
  Trip Signal : Outport
  iq : Outport  Port=2
  wires:
  Duration of Vmag<Vth/1 -> Discrete-Time Integrator1/2, Discrete-Time Integrator1/1
  GreaterThan/1 -> Trip Signal/1
  Discrete-Time Integrator1/1 -> GreaterThan/1
  Vmag vs Trip time/1 -> GreaterThan/2
  Vmag vs iq/1 -> Saturation2/1
  Gain1/1 -> iq/1
  Saturation2/1 -> Gain1/1
  Vmag/1 -> Vmag vs iq/1, Vmag vs Trip time/1, Duration of Vmag<Vth/1

== system HVDCMTGW/Wind Farm 2/Wind Farm/Detail/Wind Farm3/Voltage VAR Control & LVRT, FRT/Voltage Control ==
  In1 : Inport
  In2 : Inport  Port=2
  Constant2 : Constant  Value=0
  Gain : Gain  Gain=windController.mv
  Sum2 : Sum  Inputs=|+-
  Switch1 : Switch  Threshold=.9  SaturateOnIntegerOverflow=off  InputSameDT=off
  Out1 : Outport
  wires:
  Gain/1 -> Out1/1
  Sum2/1 -> Switch1/1
  Switch1/1 -> Gain/1
  In1/1 -> Sum2/2, Switch1/2
  Constant2/1 -> Switch1/3
  In2/1 -> Sum2/1

== system HVDCMTGW/Wind Farm 1/Wind Farm/Abstract/Wind Farm2/Voltage VAR Control & LVRT, FRT/Frequency RideThrough/Avoid Operation ==
  f_in : Inport
  Constant : Constant  Value=grid.frequency  SampleTime=Ts
  Step : Step  Time=0.5  SampleTime=Ts
  Switch : Switch  Criteria=u2 > Threshold  SaturateOnIntegerOverflow=off  InputSameDT=off
  f : Outport
  wires:
  f_in/1 -> Switch/1
  Constant/1 -> Switch/3
  Step/1 -> Switch/2
  Switch/1 -> f/1

== system HVDCMTGW/Wind Farm 1/Wind Farm/Detail/Wind Farm1/Voltage VAR Control & LVRT, FRT/Frequency RideThrough/Avoid Operation ==
  f_in : Inport
  Constant : Constant  Value=grid.frequency  SampleTime=Ts
  Step : Step  Time=0.5  SampleTime=Ts
  Switch : Switch  Criteria=u2 > Threshold  SaturateOnIntegerOverflow=off  InputSameDT=off
  f : Outport
  wires:
  f_in/1 -> Switch/1
  Constant/1 -> Switch/3
  Step/1 -> Switch/2
  Switch/1 -> f/1

== system HVDCMTGW/Wind Farm 1/Wind Farm/Detail/Wind Farm2/Voltage VAR Control & LVRT, FRT/Frequency RideThrough/Avoid Operation ==
  f_in : Inport
  Constant : Constant  Value=grid.frequency  SampleTime=Ts
  Step : Step  Time=0.5  SampleTime=Ts
  Switch : Switch  Criteria=u2 > Threshold  SaturateOnIntegerOverflow=off  InputSameDT=off
  f : Outport
  wires:
  f_in/1 -> Switch/1
  Constant/1 -> Switch/3
  Step/1 -> Switch/2
  Switch/1 -> f/1

== system HVDCMTGW/Wind Farm 1/Wind Farm/Detail/Wind Farm3/Voltage VAR Control & LVRT, FRT/Frequency RideThrough/Avoid Operation ==
  f_in : Inport
  Constant : Constant  Value=grid.frequency  SampleTime=Ts
  Step : Step  Time=0.5  SampleTime=Ts
  Switch : Switch  Criteria=u2 > Threshold  SaturateOnIntegerOverflow=off  InputSameDT=off
  f : Outport
  wires:
  f_in/1 -> Switch/1
  Constant/1 -> Switch/3
  Step/1 -> Switch/2
  Switch/1 -> f/1

== system HVDCMTGW/Wind Farm 2/Wind Farm/Abstract/Wind Farm2/Voltage VAR Control & LVRT, FRT/Frequency RideThrough/Avoid Operation ==
  f_in : Inport
  Constant : Constant  Value=grid.frequency  SampleTime=Ts
  Step : Step  Time=0.5  SampleTime=Ts
  Switch : Switch  Criteria=u2 > Threshold  SaturateOnIntegerOverflow=off  InputSameDT=off
  f : Outport
  wires:
  f_in/1 -> Switch/1
  Constant/1 -> Switch/3
  Step/1 -> Switch/2
  Switch/1 -> f/1

== system HVDCMTGW/Wind Farm 2/Wind Farm/Detail/Wind Farm1/Voltage VAR Control & LVRT, FRT/Frequency RideThrough/Avoid Operation ==
  f_in : Inport
  Constant : Constant  Value=grid.frequency  SampleTime=Ts
  Step : Step  Time=0.5  SampleTime=Ts
  Switch : Switch  Criteria=u2 > Threshold  SaturateOnIntegerOverflow=off  InputSameDT=off
  f : Outport
  wires:
  f_in/1 -> Switch/1
  Constant/1 -> Switch/3
  Step/1 -> Switch/2
  Switch/1 -> f/1

== system HVDCMTGW/Wind Farm 2/Wind Farm/Detail/Wind Farm2/Voltage VAR Control & LVRT, FRT/Frequency RideThrough/Avoid Operation ==
  f_in : Inport
  Constant : Constant  Value=grid.frequency  SampleTime=Ts
  Step : Step  Time=0.5  SampleTime=Ts
  Switch : Switch  Criteria=u2 > Threshold  SaturateOnIntegerOverflow=off  InputSameDT=off
  f : Outport
  wires:
  f_in/1 -> Switch/1
  Constant/1 -> Switch/3
  Step/1 -> Switch/2
  Switch/1 -> f/1

== system HVDCMTGW/Wind Farm 2/Wind Farm/Detail/Wind Farm3/Voltage VAR Control & LVRT, FRT/Frequency RideThrough/Avoid Operation ==
  f_in : Inport
  Constant : Constant  Value=grid.frequency  SampleTime=Ts
  Step : Step  Time=0.5  SampleTime=Ts
  Switch : Switch  Criteria=u2 > Threshold  SaturateOnIntegerOverflow=off  InputSameDT=off
  f : Outport
  wires:
  f_in/1 -> Switch/1
  Constant/1 -> Switch/3
  Step/1 -> Switch/2
  Switch/1 -> f/1
